simulink subsystem "SelfDefined_Full_Bridge_Converter"  (R2024b)
settings: Solver=VariableStepAuto  StartTime=0.0  StopTime=10.0  RelTol=1e-3
libraries: spsIGBTDiodeLib x4, simulink x1
settings Model: Creator=XixiLab  LastModifiedBy=XixiLab

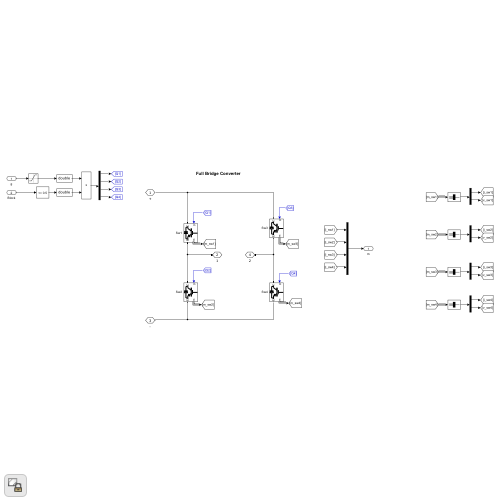
[thumbnail: Simulink's stored preview of the top-level diagram]
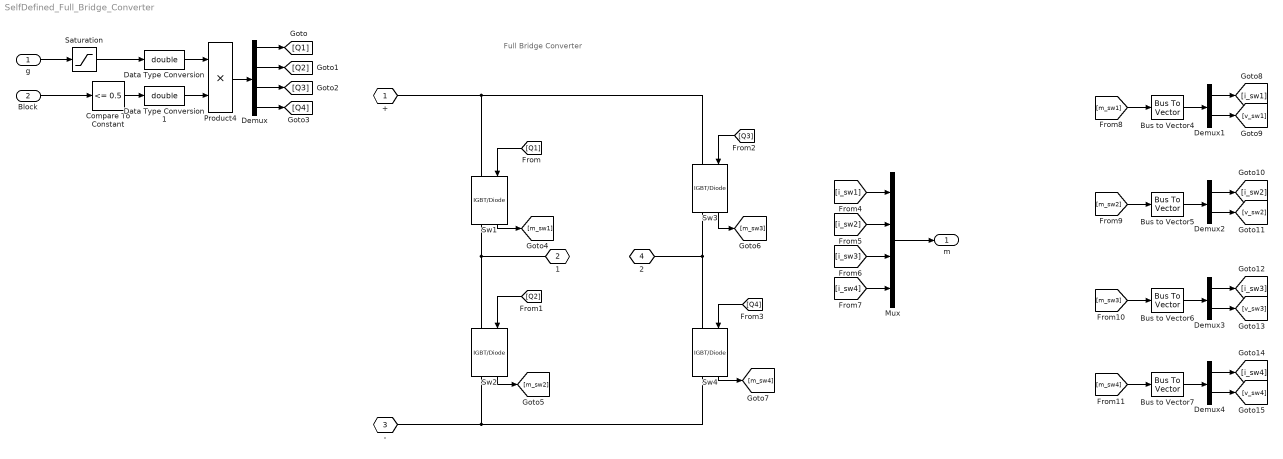
== system SelfDefined_Full_Bridge_Converter ==
  note: Full Bridge Converter
  g : Inport  PortDimensions=4
  Block : Inport  Port=2  PortDimensions=1
  Bus to Vector{4..7} (4 alike) : BusToVector
  Compare To Constant : simulink/Logic and Bit Operations/Compare To Constant  relop=<=  const=0.5  OutDataTypeStr=boolean
  Data Type Conversion : DataTypeConversion  OutDataTypeStr=double  SaturateOnIntegerOverflow=off  RndMeth=Floor
  Data Type Conversion1 : DataTypeConversion  OutDataTypeStr=double  SaturateOnIntegerOverflow=off  RndMeth=Floor
  Demux : Demux
  Demux{1..4} (4 alike) : Demux  Outputs=2
  Mux : Mux
  Product4 : Product
  Saturation : Saturate  UpperLimit=1  LowerLimit=0
  Sw{1..4} (4 alike) : spsIGBTDiodeLib/IGBT//Diode  Ron=1e-3  Rs=1e6  Cs=inf  Measurements=on
  + : PMIOPort  Tag=PMCPort  Side=Right
  1 : PMIOPort  Tag=PMCPort  Port=2  Side=Left
  - : PMIOPort  Tag=PMCPort  Port=3  Side=Right
  2 : PMIOPort  Tag=PMCPort  Port=4  Side=Left
  m : Outport
  wires:
  [Q4] -> Sw4/1
  Demux/3 -> [Q3]
  Product4/1 -> Demux/1
  Demux/2 -> [Q2]
  [Q2] -> Sw2/1
  Data Type Conversion/1 -> Product4/1
  Demux/4 -> [Q4]
  g/1 -> Saturation/1
  Saturation/1 -> Data Type Conversion/1
  Compare To Constant/1 -> Data Type Conversion1/1
  Block/1 -> Compare To Constant/1
  [Q3] -> Sw3/1
  Data Type Conversion1/1 -> Product4/2
  Demux/1 -> [Q1]
  [Q1] -> Sw1/1
  Sw1/1 -> [m_sw1]
  Sw2/1 -> [m_sw2]
  Sw3/1 -> [m_sw3]
  Sw4/1 -> [m_sw4]
  Mux/1 -> m/1
  [m_sw3] -> Bus to Vector6/1
  [m_sw2] -> Bus to Vector5/1
  Bus to Vector4/1 -> Demux1/1
  [m_sw1] -> Bus to Vector4/1
  [m_sw4] -> Bus to Vector7/1
  Demux1/1 -> [i_sw1]
  Demux1/2 -> [v_sw1]
  Demux2/2 -> [v_sw2]
  Bus to Vector5/1 -> Demux2/1
  Demux2/1 -> [i_sw2]
  Bus to Vector6/1 -> Demux3/1
  Demux3/1 -> [i_sw3]
  Demux3/2 -> [v_sw3]
  Bus to Vector7/1 -> Demux4/1
  Demux4/1 -> [i_sw4]
  Demux4/2 -> [v_sw4]
  [i_sw1] -> Mux/1
  [i_sw2] -> Mux/2
  [i_sw3] -> Mux/3
  [i_sw4] -> Mux/4
  connections:
  Sw2/RConn1 -- -/RConn1 -- Sw4/RConn1
  Sw1/LConn1 -- +/RConn1 -- Sw3/LConn1
  Sw3/RConn1 -- 2/RConn1 -- Sw4/LConn1
  Sw1/RConn1 -- 1/RConn1 -- Sw2/LConn1
